simulink library "SumDBSPL"  (R2022b)
settings: Solver=VariableStepAuto  StartTime=0.0  StopTime=10.0  RelTol=1e-3
settings Model: Creator=bt1030690  LastModifiedBy=kl13806
settings SolverCC: AlgebraicLoopSolver=TrustRegion
settings DebuggingCC: UnconnectedInputMsg=warning  UnconnectedOutputMsg=warning  UnconnectedLineMsg=warning  SFMachineParentedDataDiag=warning  ArithmeticOperatorsInVariantConditions=warning
settings ModelReferenceCC: EnableRefExpFcnMdlSchedulingChecks=on
settings SFSimCC: SimUseLocalCustomCode=off  CustomCodeUndefinedFunction=UseInterfaceOnly
settings RTWCC: RTWUseLocalCustomCode=off  DLArmComputeVersion=19.05
settings CodeAppCC: StateflowObjectComments=on

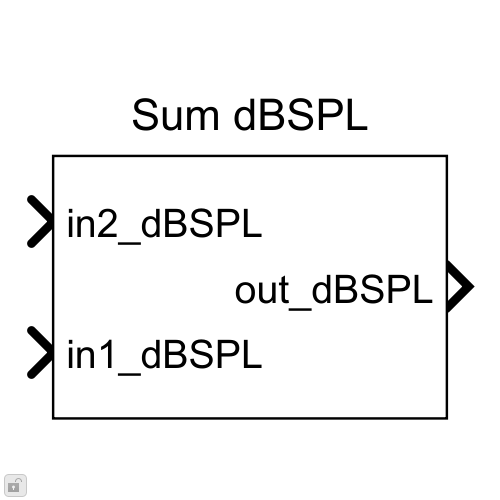
[thumbnail: Simulink's stored preview of the top-level diagram]
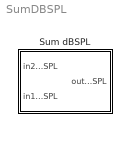
== system SumDBSPL ==
  Sum dBSPL : Subsystem

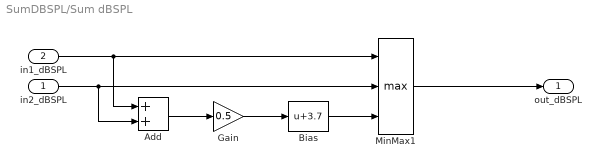
== system SumDBSPL/Sum dBSPL ==
  in2_dBSPL : Inport
  in1_dBSPL : Inport  Port=2
  Add : Sum
  Bias : Bias  Bias=3.7  SaturateOnIntegerOverflow=off
  Gain : Gain  Gain=0.5
  MinMax1 : MinMax  Function=max  Inputs=3
  out_dBSPL : Outport
  wires:
  in1_dBSPL/1 -> MinMax1/1, Add/1
  in2_dBSPL/1 -> MinMax1/2, Add/2
  MinMax1/1 -> out_dBSPL/1
  Add/1 -> Gain/1
  Gain/1 -> Bias/1
  Bias/1 -> MinMax1/3
